simulink model "AFASClosedloopSim"  (R2023a)
settings: Solver=FixedStepAuto  StartTime=0.0  StopTime=600  FixedStep=1/240  RelTol=1e-5
PreLoadFcn:
  | [aircraft, state] = astDehavillandBeaver();
  | thrustX = getCoefficient(aircraft,"CX","Propeller",Component="Propeller");
InitFcn:
  | AFASClosedloopSimInitialization
model workspace (MATLAB code in the model file + MAT data in the model file):
  AirReferencedVelocity = 1
  AircraftPerformance : object (value not decoded)
  CurrentWaypoint = 1
  FCCLatDirMode = 1
  FCCVerticalMode = 1
  FlightPlan = 1
  LookaheadDis = 15
  NextWaypoint = 1
  NumofWaypoint = 1
  OwnshipAircraftID = 1
  PreWaypoint = 1
  PreviousWaypoint : Simulink.Parameter (value not decoded)
  TrajectoryChange = 1
  WaypointType = 1
  inputs0 : object (value not decoded)
  states : object (value not decoded)
  states0 : object (value not decoded)
  other statements: initialize6DOFSkyHogg;
values from neighbouring files (symbols this model uses):
  alt_ft = 1000    [AFASClosedloopSimInitialization.m]
  alt_hold_av = 1.5    [AFASClosedloopSimInitialization.m]
  alt_hold_hold = 0.1    [AFASClosedloopSimInitialization.m]
  alt_hold_vs = 0.58    [AFASClosedloopSimInitialization.m]
  alt_m = 304.8    [AFASClosedloopSimInitialization.m]
  AT_lead_T1 = 1    [AFASClosedloopSimInitialization.m]
  AT_lead_T2 = 1    [AFASClosedloopSimInitialization.m]
  AT_spd_hold_cmpst = 0.5    [AFASClosedloopSimInitialization.m]
  AT_spd_hold_ptch_tau_gain = 0.15    [AFASClosedloopSimInitialization.m]
  AT_spd_hold_rate_damping_gain = 10    [AFASClosedloopSimInitialization.m]
  AT_spd_hold_tas_lp_tau = 5.0    (= 5)    [AFASClosedloopSimInitialization.m]
  AT_spd_hold_tas_val_lp_tau = 0.5    [AFASClosedloopSimInitialization.m]
  AT_struct_den = 1    [AFASClosedloopSimInitialization.m]
  AT_struct_num = 1    [AFASClosedloopSimInitialization.m]
  AT_svo_composite = 1    [AFASClosedloopSimInitialization.m]
  av_hp_fltr_tau = 10    [AFASClosedloopSimInitialization.m]
  av_lp_fltr_tau = 0.5    [AFASClosedloopSimInitialization.m]
  cas_mps = 72.0222    [AFASClosedloopSimInitialization.m]
  Cl0 = 5.910000000000000e-04    (= 0.000591)    [AFASClosedloopSimInitialization.m]
  Cl_beta = -0.0618    [AFASClosedloopSimInitialization.m]
  Cl_da = -0.0992    [AFASClosedloopSimInitialization.m]
  Cl_da_alpha = -0.0827    [AFASClosedloopSimInitialization.m]
  Cl_dr = 0.0069    [AFASClosedloopSimInitialization.m]
  Cl_p = -0.5045    [AFASClosedloopSimInitialization.m]
  Cl_r = 0.1695    [AFASClosedloopSimInitialization.m]
  Cm0 = 0.0945    [AFASClosedloopSimInitialization.m]
  Cm_alpha = -0.6028    [AFASClosedloopSimInitialization.m]
  Cm_alpha2 = -2.1400    (= -2.14)    [AFASClosedloopSimInitialization.m]
  Cm_beta2 = 0.6921    [AFASClosedloopSimInitialization.m]
  Cm_de = -1.9210    (= -1.921)    [AFASClosedloopSimInitialization.m]
  Cm_df = 0.4072    [AFASClosedloopSimInitialization.m]
  Cm_q = -15.5600    (= -15.56)    [AFASClosedloopSimInitialization.m]
  Cm_r = -0.3118    [AFASClosedloopSimInitialization.m]
  Cn0 = -0.0031    [AFASClosedloopSimInitialization.m]
  Cn_beta = 0.0067    [AFASClosedloopSimInitialization.m]
  Cn_beta3 = 0.1373    [AFASClosedloopSimInitialization.m]
  Cn_da = -0.0039    [AFASClosedloopSimInitialization.m]
  Cn_dr = -0.0827    [AFASClosedloopSimInitialization.m]
  Cn_p = -0.1585    [AFASClosedloopSimInitialization.m]
  Cn_q = 0.1595    [AFASClosedloopSimInitialization.m]
  Cn_r = -0.1112    [AFASClosedloopSimInitialization.m]
  Cx0 = -0.0355    [AFASClosedloopSimInitialization.m]
  Cx_alpha = 0.0029    [AFASClosedloopSimInitialization.m]
  Cx_alpha2 = 5.4590    (= 5.459)    [AFASClosedloopSimInitialization.m]
  Cx_alpha3 = -5.1620    (= -5.162)    [AFASClosedloopSimInitialization.m]
  Cx_df = -0.0945    [AFASClosedloopSimInitialization.m]
  Cx_df_alpha = 1.1060    (= 1.106)    [AFASClosedloopSimInitialization.m]
  Cx_dr = 0.0341    [AFASClosedloopSimInitialization.m]
  Cx_q = -0.6748    [AFASClosedloopSimInitialization.m]
  Cy0 = -0.0022    [AFASClosedloopSimInitialization.m]
  Cy_beta = -0.7678    [AFASClosedloopSimInitialization.m]
  Cy_da = -0.0296    [AFASClosedloopSimInitialization.m]
  Cy_dr = 0.1158    [AFASClosedloopSimInitialization.m]
  Cy_dr_alpha = 0.5238    [AFASClosedloopSimInitialization.m]
  Cy_p = -0.1240    (= -0.124)    [AFASClosedloopSimInitialization.m]
  Cy_r = 0.3666    [AFASClosedloopSimInitialization.m]
  Cz0 = -0.0550    (= -0.055)    [AFASClosedloopSimInitialization.m]
  Cz_alpha = -5.5780    (= -5.578)    [AFASClosedloopSimInitialization.m]
  Cz_alpha3 = 3.4420    (= 3.442)    [AFASClosedloopSimInitialization.m]
  Cz_de = -0.3980    (= -0.398)    [AFASClosedloopSimInitialization.m]
  Cz_de_beta = -15.9300    (= -15.93)    [AFASClosedloopSimInitialization.m]
  Cz_df = -1.3770    (= -1.377)    [AFASClosedloopSimInitialization.m]
  Cz_df_alpha = -1.2610    (= -1.261)    [AFASClosedloopSimInitialization.m]
  Cz_q = -2.9880    (= -2.988)    [AFASClosedloopSimInitialization.m]
  hdg_select_hdg_rate_capt = 0.2    [AFASClosedloopSimInitialization.m]
  hdg_select_hdg_rate_damping = 1    [AFASClosedloopSimInitialization.m]
  hdg_select_hdg_rate_track = 0.05    [AFASClosedloopSimInitialization.m]
  lat_accel_aug_lp_tau = 10    [AFASClosedloopSimInitialization.m]
  ltrl_acc_gain = -0.04    [AFASClosedloopSimInitialization.m]
  ltrl_acc_lp_tau = 0.5    [AFASClosedloopSimInitialization.m]
  mach = 0.213    [AFASClosedloopSimInitialization.m]
  OwnshipAircraftConfig = 0    [AFASClosedloopSimInitialization.m]
  pitch_att_gain = 0.7    [AFASClosedloopSimInitialization.m]
  pitch_lead_T1 = 1    [AFASClosedloopSimInitialization.m]
  pitch_lead_T2 = 1    [AFASClosedloopSimInitialization.m]
  pitch_rate_gain = -1400    [AFASClosedloopSimInitialization.m]
  pitch_rate_gain_GAIN1 = -56    [AFASClosedloopSimInitialization.m]
  pitch_rate_gain_GAIN2 = -52.25    [AFASClosedloopSimInitialization.m]
  pitch_rate_gain_IAS1 = 100    [AFASClosedloopSimInitialization.m]
  pitch_rate_gain_IAS2 = 380    [AFASClosedloopSimInitialization.m]
  pitch_rate_gain_schd = [4.24        2.80        2.24        1.68        1.44        1.22        0.97        0.85        0.77        0.72        0.66    ] * 1000    [AFASClosedloopSimInitialization.m]
  pitch_rate_gain_spd = [85          100.0       120.00      140.00      160.00      180.00      200.00      220.00      240.00      260.00      275.00  ] * 0.5144444    [AFASClosedloopSimInitialization.m]
  pitch_schedule_type = 3    [AFASClosedloopSimInitialization.m]
  pitch_struct_den = 1    [AFASClosedloopSimInitialization.m]
  pitch_struct_num = 1    [AFASClosedloopSimInitialization.m]
  pitch_svo_composite = 1    [AFASClosedloopSimInitialization.m]
  pitch_svo_integral = 0.6    [AFASClosedloopSimInitialization.m]
  roll_att_gain = 0.45    [AFASClosedloopSimInitialization.m]
  roll_lead_T1 = 1    [AFASClosedloopSimInitialization.m]
  roll_lead_T2 = 1    [AFASClosedloopSimInitialization.m]
  roll_limit = 30*d2r    (= 0.5235987)    [AFASClosedloopSimInitialization.m]
  roll_rate_gain = 561.5    [AFASClosedloopSimInitialization.m]
  roll_rate_gain_GAIN1 = 57.25    [AFASClosedloopSimInitialization.m]
  roll_rate_gain_GAIN2 = 41.25    [AFASClosedloopSimInitialization.m]
  roll_rate_gain_IAS1 = 100    [AFASClosedloopSimInitialization.m]
  roll_rate_gain_IAS2 = 380    [AFASClosedloopSimInitialization.m]
  roll_rate_gain_schd = [1.30        0.86        0.71        0.63        0.57        0.50        0.46        0.46    ] * 1000    [AFASClosedloopSimInitialization.m]
  roll_rate_gain_spd = [85.00       100.00      120.00      140.00      160.00      200.00      220.00      275.00  ] * 0.5144444    [AFASClosedloopSimInitialization.m]
  roll_schedule_type = 3    [AFASClosedloopSimInitialization.m]
  roll_struct_den = 1    [AFASClosedloopSimInitialization.m]
  roll_struct_num = 1    [AFASClosedloopSimInitialization.m]
  roll_svo_composite = 0.00001    (= 1e-05)    [AFASClosedloopSimInitialization.m]
  roll_svo_integral = 0.6    [AFASClosedloopSimInitialization.m]
  tas_mps = 73.051    [AFASClosedloopSimInitialization.m]
  TGR = 0.25    [AFASClosedloopSimInitialization.m]
  wingrock_enable_alt = 20000    [AFASClosedloopSimInitialization.m]
  wingrock_enable_mach = 0.6    [AFASClosedloopSimInitialization.m]
  wingrock_lookup_data = [2 2  1 1]    [AFASClosedloopSimInitialization.m]
  wingrock_lookup_row = [0 2 5 10]*pi/180    [AFASClosedloopSimInitialization.m]
  wingrock_schedule_type = 3    [AFASClosedloopSimInitialization.m]
  yaw_rate_gain = 15521    [AFASClosedloopSimInitialization.m]
  yaw_rate_gain_GAIN1 = 37.8352    [AFASClosedloopSimInitialization.m]
  yaw_rate_gain_GAIN2 = 24.2654    [AFASClosedloopSimInitialization.m]
  yaw_rate_gain_IAS1 = 100    [AFASClosedloopSimInitialization.m]
  yaw_rate_gain_IAS2 = 340    [AFASClosedloopSimInitialization.m]
  yaw_rate_gain_piecewise_schd = [7.68	5.98		3.22	2.59		1.78 ... (first row only)    [AFASClosedloopSimInitialization.m]
  yaw_rate_gain_schd = [15521    11532   11532   10115   8951.7  7831.7  6829.2  5739.3  4506.7  3317.9  3391.5  2103.9  1404.5  994.3226]    [AFASClosedloopSimInitialization.m]
  yaw_rate_gain_spd = [90       97      106     111     118     127     136     149     165     187     192     228     264     295     ] * 0.5144444    [AFASClosedloopSimInitialization.m]
  yaw_rate_hp_tau = 1.8    [AFASClosedloopSimInitialization.m]
  yd_lead_T1 = yd_a * yd_lead_T2    [AFASClosedloopSimInitialization.m]
  ... (+7 more)
undefined symbols (not defined in the file or in its folder): aircraft, DiscIntNeverNeededParam, Earth, F, Light, MIL, sigbuilder_block, state, WGS84
libraries: aerolibasang x4, aerolibactuator x4, aerolibguid x2, simulink x2, dspnetwork x2, etargetslib x2, shared6dof x1, aerolibadyn x1, aerolibatmos2 x1, aerolibwind2 x1, aerolibtransform2 x1, sharedtransform x1
(part 3 of 4)

== system AFASClosedloopSim/FMGC (Flight Mgt and Guidance & Control)/AFCC: Albatross.ai Flight Control Computer/FCC: Outerloop & Innerloop Control Laws ==
  SpdTargetLimited : Inport
  AltTargetLimited : Inport  Port=2
  HDGTargetLimited : Inport  Port=3
  OwnshipStates : Inport  Port=4
  ALT Mode : Subsystem
  Autothrottle : Subsystem
  HDG Mode : Subsystem
  ATServoCmd : Outport
  PitchServoCmd : Outport  Port=2
  RollSevoCmd : Outport  Port=3
  YawServoCmd : Outport  Port=4
  wires:
  Autothrottle/1(ATServoCmd) -> ATServoCmd/1
  SpdTargetLimited/1 -> Autothrottle/1(SpeedTargetLimited)
  AltTargetLimited/1 -> ALT Mode/1(AltTargetLimited)
  OwnshipStates/1 -> HDG Mode/2(OwnshipStates), ALT Mode/2(OwnshipStates), Autothrottle/2(OwnshipStates)
  HDGTargetLimited/1 -> HDG Mode/1(HDGTargetLimited)
  ALT Mode/1(motorPosCmd_rad) -> PitchServoCmd/1
  HDG Mode/1(ailMotorPosCmd_rad) -> RollSevoCmd/1
  HDG Mode/2(rudMotorPosCmd_rad) -> YawServoCmd/1

== system AFASClosedloopSim/FMGC (Flight Mgt and Guidance & Control)/AFMS: Albatross Flight Management System/WGS84_Location ==
  lon : Inport
  lat : Inport  Port=2
  alt : Inport  Port=3
  C Caller : CCaller  FunctionName=latToMeters  PortSpecificationStruct="%)30     .    6 4   8    (     @         %    \"     ,    !     0         %  0 \"0    $    _    07)G3F%M90  4&]R=$YA;64 4V-O<&4     26YD97@     5'EP90      4VEZ90      27-';&]B86P   X    P    !@    @    $          4    (     0    ,    !         !   P!O=70 #@   #     &    \"     0         !0    @    !     P    $         $  # &]U=  .    .     8    (    !          %    \"     $    &     0         0    !@   $]U='!U=   #@   #@    &    \"     8         !0    @    !     0    $         \"0    @               X    X    !@    @    $          4    (     0    8    !         !     &    9&]U8FQE   .    ,     8    (    !          %    \"     $    !     0         0  $ ,0    X    P    !@    @    ) @        4    (     0    $    !          (  0      #@   #     &    \"     0         !0    @    !    !     $         $  $ &QA=#$.    ,     8    (    !          %    \"     $    $     0         0  0 ;&%T,0X    X    !@    @    $          4    (     0    4    !         !     %    26YP=70    .    .     8    (    !@         %    \"     $    !     0         )    \"               #@   #@    &    \"     0         !0    @    !    !@    $         $     8   !D;W5B;&4   X    P    !@    @    $          4    (     0    $    !         !   0 Q    #@   #     &    \"     D\"        !0    @    !     0    $          @ !       .    ,     8    (    !          %    \"     $    $     0         0  0 ;&%T,@X    P    !@    @    $          4    (     0    0    !         !  ! !L870R#@   #@    &    \"     0         !0    @    !    !0    $         $     4   !);G!U=     X    X    !@    @    &          4    (     0    $    !          D    (            \\#\\.    .     8    (    !          %    \"     $    &     0         0    !@   &1O=6)L90  #@   #     &    \"     0         !0    @    !     0    $         $  ! #$    .    ,     8    (    \"0(        %    \"     $    !     0         \"  $"
  C Caller1 : CCaller  FunctionName=lonToMeters  PortSpecificationStruct="%)30     .    ^ 8   8    (     @         %    \"     0    !     0         %  0 \"0    $    _    07)G3F%M90  4&]R=$YA;64 4V-O<&4     26YD97@     5'EP90      4VEZ90      27-';&]B86P   X    P    !@    @    $          4    (     0    ,    !         !   P!O=70 #@   #     &    \"     0         !0    @    !     P    $         $  # &]U=  .    .     8    (    !          %    \"     $    &     0         0   ...(+2020 chars)"
  lat1 : Constant  Value=39.13730579607521
  lon1 : Constant  Value=117.33825437858884
  x : Outport
  y : Outport  Port=2
  z : Outport  Port=3
  wires:
  lon1/1 -> C Caller1/2
  lon/1 -> C Caller1/1
  alt/1 -> z/1
  lat1/1 -> C Caller/2, C Caller1/3
  lat/1 -> C Caller/1
  C Caller/1 -> y/1
  C Caller1/1 -> x/1

== system AFASClosedloopSim/6 DoF Airframe Model/Aerodynamic Model/Actuator Increments/Aileron ==
  alpha : Inport  Unit=rad
  Actuators : Inport  Port=2  Unit=rad
  Gain1 : Gain  Gain=0  SaturateOnIntegerOverflow=on  OutDataTypeStr=Inherit: Same as input  ParamDataTypeStr=Inherit: Same as input
  Gain2 : Gain  Gain=Cy_da  SaturateOnIntegerOverflow=on  OutDataTypeStr=Inherit: Same as input  ParamDataTypeStr=Inherit: Same as input
  Gain3 : Gain  Gain=0  SaturateOnIntegerOverflow=on  OutDataTypeStr=Inherit: Same as input  ParamDataTypeStr=Inherit: Same as input
  Gain4 : Gain  Gain=Cn_da  SaturateOnIntegerOverflow=on  OutDataTypeStr=Inherit: Same as input  ParamDataTypeStr=Inherit: Same as input
  Gain5 : Gain  Gain=0  SaturateOnIntegerOverflow=on  OutDataTypeStr=Inherit: Same as input  ParamDataTypeStr=Inherit: Same as input
  Gain6 : Gain  Gain=Cl_da  SaturateOnIntegerOverflow=on  OutDataTypeStr=Inherit: Same as input  ParamDataTypeStr=Inherit: Same as input
  Gain7 : Gain  Gain=Cl_da_alpha  SaturateOnIntegerOverflow=on  OutDataTypeStr=Inherit: Same as input  ParamDataTypeStr=Inherit: Same as input
  Mux1 : Mux  Inputs=6
  Product4 : Product  InputSameDT=on  SaturateOnIntegerOverflow=on  OutDataTypeStr=Inherit: Same as first input
  Selector1 : Selector  IndexMode=Zero-based  InputPortWidth=4  IndexOptions=Index vector (dialog)  Indices=1  OutputSizes=1
  Sum1 : Sum  Inputs=++|  SaturateOnIntegerOverflow=on
  delCoeff : Outport  VectorParamsAs1DForOutWhenUnconnected=off
  wires:
  Gain6/1 -> Sum1/1
  Sum1/1 -> Mux1/4
  Gain7/1 -> Sum1/2
  Product4/1 -> Gain7/1
  Gain1/1 -> Mux1/1  "Cx"
  alpha/1 -> Product4/2
  Actuators/1 -> Selector1/1
  Mux1/1 -> delCoeff/1
  Gain2/1 -> Mux1/2  "Cy"
  Gain3/1 -> Mux1/3  "Cz"
  Gain5/1 -> Mux1/5  "Cm"
  Gain4/1 -> Mux1/6
  Selector1/1 -> Gain1/1, Gain2/1, Gain3/1, Gain6/1, Product4/1, Gain5/1, Gain4/1

== system AFASClosedloopSim/6 DoF Airframe Model/Aerodynamic Model/Actuator Increments/Elevator ==
  Actuators : Inport
  Beta : Inport  Port=2  Unit=rad
  Constant1 : Constant  Value=0
  Gain1 : Gain  Gain=Cz_de  SaturateOnIntegerOverflow=on  OutDataTypeStr=Inherit: Same as input  ParamDataTypeStr=Inherit: Same as input
  Gain2 : Gain  Gain=Cz_de_beta  SaturateOnIntegerOverflow=on  OutDataTypeStr=Inherit: Same as input  ParamDataTypeStr=Inherit: Same as input
  Gain3 : Gain  Gain=Cm_de  SaturateOnIntegerOverflow=on  OutDataTypeStr=Inherit: Same as input  ParamDataTypeStr=Inherit: Same as input
  Mux1 : Mux  Inputs=6
  Product4 : Product  Inputs=3  InputSameDT=on  SaturateOnIntegerOverflow=on  OutDataTypeStr=Inherit: Same as first input
  Selector1 : Selector  IndexMode=Zero-based  InputPortWidth=4  IndexOptions=Index vector (dialog)  Indices=0  OutputSizes=1
  Sum1 : Sum  SaturateOnIntegerOverflow=on
  delCoeff : Outport  VectorParamsAs1DForOutWhenUnconnected=off
  wires:
  Gain3/1 -> Mux1/5
  Gain1/1 -> Sum1/2
  Gain2/1 -> Sum1/1
  Sum1/1 -> Mux1/3
  Product4/1 -> Gain2/1
  Beta/1 -> Product4/2, Product4/1
  Mux1/1 -> delCoeff/1
  Selector1/1 -> Gain3/1, Gain1/1, Product4/3
  Constant1/1 -> Mux1/1, Mux1/2, Mux1/4, Mux1/6
  Actuators/1 -> Selector1/1

== system AFASClosedloopSim/6 DoF Airframe Model/Aerodynamic Model/Actuator Increments/Flap ==
  Alpha : Inport  Unit=rad
  Actuators : Inport  Port=2  Unit=rad
  Constant1 : Constant  Value=0
  Constant2 : Constant  Value=0
  Constant3 : Constant  Value=0
  Gain1 : Gain  Gain=Cx_df  SaturateOnIntegerOverflow=on  OutDataTypeStr=Inherit: Same as input  ParamDataTypeStr=Inherit: Same as input
  Gain2 : Gain  Gain=Cx_df_alpha  SaturateOnIntegerOverflow=on  OutDataTypeStr=Inherit: Same as input  ParamDataTypeStr=Inherit: Same as input
  Gain3 : Gain  Gain=Cz_df  SaturateOnIntegerOverflow=on  OutDataTypeStr=Inherit: Same as input  ParamDataTypeStr=Inherit: Same as input
  Gain4 : Gain  Gain=Cz_df_alpha  SaturateOnIntegerOverflow=on  OutDataTypeStr=Inherit: Same as input  ParamDataTypeStr=Inherit: Same as input
  Gain5 : Gain  Gain=Cm_df  SaturateOnIntegerOverflow=on  OutDataTypeStr=Inherit: Same as input  ParamDataTypeStr=Inherit: Same as input
  Mux1 : Mux  Inputs=6
  Product1 : Product  InputSameDT=on  SaturateOnIntegerOverflow=on  OutDataTypeStr=Inherit: Same as first input
  Product4 : Product  InputSameDT=on  SaturateOnIntegerOverflow=on  OutDataTypeStr=Inherit: Same as first input
  Selector1 : Selector  IndexMode=Zero-based  InputPortWidth=4  IndexOptions=Index vector (dialog)  Indices=3  OutputSizes=1
  Sum1 : Sum  SaturateOnIntegerOverflow=on
  Sum2 : Sum  SaturateOnIntegerOverflow=on
  delCoeff : Outport  VectorParamsAs1DForOutWhenUnconnected=off
  wires:
  Selector1/1 -> Gain1/1, Product4/1, Product1/1, Gain3/1, Gain5/1
  Actuators/1 -> Selector1/1
  Gain5/1 -> Mux1/5
  Gain3/1 -> Sum2/1
  Gain4/1 -> Sum2/2
  Product1/1 -> Gain4/1
  Gain1/1 -> Sum1/1
  Gain2/1 -> Sum1/2
  Product4/1 -> Gain2/1
  Alpha/1 -> Product1/2, Product4/2
  Mux1/1 -> delCoeff/1
  Sum1/1 -> Mux1/1
  Sum2/1 -> Mux1/3
  Constant1/1 -> Mux1/2
  Constant2/1 -> Mux1/4
  Constant3/1 -> Mux1/6

== system AFASClosedloopSim/6 DoF Airframe Model/Aerodynamic Model/Actuator Increments/Rudder ==
  Alpha : Inport  Unit=rad
  Actuators : Inport  Port=2  Unit=rad
  Constant1 : Constant  Value=0
  Constant2 : Constant  Value=0
  Gain1 : Gain  Gain=Cl_dr  SaturateOnIntegerOverflow=on  OutDataTypeStr=Inherit: Same as input  ParamDataTypeStr=Inherit: Same as input
  Gain2 : Gain  Gain=Cn_dr  SaturateOnIntegerOverflow=on  OutDataTypeStr=Inherit: Same as input  ParamDataTypeStr=Inherit: Same as input
  Gain3 : Gain  Gain=Cy_dr_alpha  SaturateOnIntegerOverflow=on  OutDataTypeStr=Inherit: Same as input  ParamDataTypeStr=Inherit: Same as input
  Gain4 : Gain  Gain=Cy_dr  SaturateOnIntegerOverflow=on  OutDataTypeStr=Inherit: Same as input  ParamDataTypeStr=Inherit: Same as input
  Gain5 : Gain  Gain=Cx_dr  SaturateOnIntegerOverflow=on  OutDataTypeStr=Inherit: Same as input  ParamDataTypeStr=Inherit: Same as input
  Mux1 : Mux  Inputs=6
  Product1 : Product  InputSameDT=on  SaturateOnIntegerOverflow=on  OutDataTypeStr=Inherit: Same as first input
  Selector1 : Selector  IndexMode=Zero-based  InputPortWidth=4  IndexOptions=Index vector (dialog)  Indices=2  OutputSizes=1
  Sum1 : Sum  SaturateOnIntegerOverflow=on
  delCoeff : Outport  VectorParamsAs1DForOutWhenUnconnected=off
  wires:
  Gain5/1 -> Mux1/1
  Gain4/1 -> Sum1/1
  Gain3/1 -> Sum1/2
  Gain1/1 -> Mux1/4
  Gain2/1 -> Mux1/6
  Product1/1 -> Gain3/1
  Alpha/1 -> Product1/2
  Mux1/1 -> delCoeff/1
  Actuators/1 -> Selector1/1
  Sum1/1 -> Mux1/2
  Constant1/1 -> Mux1/3
  Constant2/1 -> Mux1/5
  Selector1/1 -> Gain5/1, Gain4/1, Product1/1, Gain1/1, Gain2/1

== system AFASClosedloopSim/6 DoF Airframe Model/Aerodynamic Model/Body Rate Damping/p ==
  Constant1 : Constant  Value=0
  Constant2 : Constant  Value=Cy_p
  Constant3 : Constant  Value=Cl_p
  Constant4 : Constant  Value=Cn_p
  Mux1 : Mux  Inputs=6
  delCoeff : Outport  VectorParamsAs1DForOutWhenUnconnected=off
  wires:
  Constant2/1 -> Mux1/2
  Mux1/1 -> delCoeff/1
  Constant1/1 -> Mux1/5, Mux1/3, Mux1/1
  Constant4/1 -> Mux1/6
  Constant3/1 -> Mux1/4

== system AFASClosedloopSim/6 DoF Airframe Model/Aerodynamic Model/Body Rate Damping/q ==
  Constant1 : Constant  Value=0
  Constant2 : Constant  Value=Cz_q
  Constant3 : Constant  Value=Cx_q
  Constant4 : Constant  Value=Cm_q
  Constant5 : Constant  Value=Cn_q
  Mux1 : Mux  Inputs=6
  delCoeff : Outport  VectorParamsAs1DForOutWhenUnconnected=off
  wires:
  Constant2/1 -> Mux1/3
  Constant5/1 -> Mux1/6
  Constant1/1 -> Mux1/4, Mux1/2
  Constant4/1 -> Mux1/5
  Constant3/1 -> Mux1/1
  Mux1/1 -> delCoeff/1

== system AFASClosedloopSim/6 DoF Airframe Model/Aerodynamic Model/Body Rate Damping/r ==
  Constant : Constant  Value=0
  Constant1 : Constant  Value=Cy_r
  Constant2 : Constant  Value=Cl_r
  Constant3 : Constant  Value=Cm_r
  Constant4 : Constant  Value=Cn_r
  Mux1 : Mux  Inputs=6
  delCoeff : Outport  VectorParamsAs1DForOutWhenUnconnected=off
  wires:
  Constant3/1 -> Mux1/5
  Constant1/1 -> Mux1/2
  Constant4/1 -> Mux1/6
  Constant2/1 -> Mux1/4
  Constant/1 -> Mux1/3, Mux1/1
  Mux1/1 -> delCoeff/1

== system AFASClosedloopSim/FMGC (Flight Mgt and Guidance & Control)/AFCC: Albatross.ai Flight Control Computer/FCC: Outerloop & Innerloop Control Laws/ALT Mode ==
  AltTargetLimited : Inport
  OwnshipStates : Inport  Port=2
  ADC Filters & Delays : Subsystem
  AHRS Filters & Delays : Subsystem
  Bus Selector : BusSelector  OutputSignals=Ze,q
  Derivative : Derivative
  Derivative1 : Derivative
  Innerloop Control Law : Subsystem
  Outerloop Control Law : Subsystem
  motorPosCmd_rad : Outport
  wires:
  Outerloop Control Law/1(thetaCmd_rad) -> Innerloop Control Law/1("thetaCmd_rad ")
  Outerloop Control Law/2(" qC_rps ") -> Innerloop Control Law/2(qC_rps)
  ADC Filters & Delays/1(hF_m) -> Outerloop Control Law/2(hF_m)
  AltTargetLimited/1 -> Outerloop Control Law/1(hCmd_m)
  Innerloop Control Law/1(motorPosCmd_rad) -> motorPosCmd_rad/1
  AHRS Filters & Delays/2(qF_rps) -> Outerloop Control Law/5(qF_rps)
  ADC Filters & Delays/2(hdF_mps) -> Outerloop Control Law/3(hdF_mps)
  Derivative/1 -> Derivative1/1, ADC Filters & Delays/2(hd_mps)
  Bus Selector/1 -> ADC Filters & Delays/1(h_m), Derivative/1  "<Ze>"
  AHRS Filters & Delays/1(hddF_mpss) -> Outerloop Control Law/4(hddF_mpss)
  OwnshipStates/1 -> Bus Selector/1
  Derivative1/1 -> AHRS Filters & Delays/1(hdd_mpss)
  Bus Selector/2 -> AHRS Filters & Delays/2(qb_rps)  "<q>"

== system AFASClosedloopSim/FMGC (Flight Mgt and Guidance & Control)/AFCC: Albatross.ai Flight Control Computer/FCC: Outerloop & Innerloop Control Laws/Autothrottle ==
  SpeedTargetLimited : Inport
  OwnshipStates : Inport  Port=2
  ADC Filters & Delays : Subsystem
  AT Innerloop : Subsystem
  AT SPD Hold/Select : Subsystem
  Add : Sum  Inputs=+-
  Bus Selector : BusSelector  OutputSignals=u
  Constant : Constant
  Constant1 : Constant
  Manual Switch1 : ManualSwitch
  Manual Switch2 : ManualSwitch
  g2mpss2 : Gain  Gain=AT_svo_composite  SaturateOnIntegerOverflow=on  OutDataTypeStr=Inherit: Same as input  ParamDataTypeStr=Inherit: Same as input
  ATServoCmd : Outport
  wires:
  OwnshipStates/1 -> Bus Selector/1
  AT SPD Hold/Select/1(ATCmd_rad) -> AT Innerloop/1("ATCmd_rad ")
  ADC Filters & Delays/1(vtasF_mps) -> AT SPD Hold/Select/2(vtasF_mps)
  Bus Selector/1 -> Add/2  "<u>"
  Add/1 -> g2mpss2/1
  g2mpss2/1 -> Manual Switch1/1
  AT Innerloop/1(motorPosCmd_rad) -> Manual Switch1/2
  Manual Switch1/1 -> ATServoCmd/1
  SpeedTargetLimited/1 -> Manual Switch2/1
  Manual Switch2/1 -> Add/1
  Constant/1 -> AT SPD Hold/Select/1(vtasCmd_mps)
  Constant1/1 -> ADC Filters & Delays/1(vtas_mps)

== system AFASClosedloopSim/FMGC (Flight Mgt and Guidance & Control)/AFCC: Albatross.ai Flight Control Computer/FCC: Outerloop & Innerloop Control Laws/HDG Mode ==
  HDGTargetLimited : Inport
  OwnshipStates : Inport  Port=2
  Bus Selector : BusSelector  OutputSignals=psi,phi,r,Ayb
  Derivative : Derivative
  Derivative1 : Derivative
  Filters & Delays : Subsystem
  Innerloop Control Law : Subsystem
  Outerloop Control Law : Subsystem
  ailMotorPosCmd_rad : Outport
  rudMotorPosCmd_rad : Outport  Port=2
  wires:
  Outerloop Control Law/2(phiC_rad) -> Innerloop Control Law/2(phiC_rad)
  Filters & Delays/4(phiDotF_rps) -> Outerloop Control Law/5("phiDotF_rps ")
  Outerloop Control Law/3(rC_rps) -> Innerloop Control Law/3(rC_rps)
  Bus Selector/2 -> Derivative1/1, Filters & Delays/3(phi_rad)  "<phi>"
  Outerloop Control Law/4(AyC_mpss) -> Innerloop Control Law/4(AyC_mpss)
  Innerloop Control Law/2(rudMotorPosCmd_rad) -> rudMotorPosCmd_rad/1
  Outerloop Control Law/5(phiDotC_rps) -> Innerloop Control Law/5(phidotC_rps)
  Innerloop Control Law/1(ailMotorPosCmd_rad) -> ailMotorPosCmd_rad/1
  Filters & Delays/3(phiF_rad) -> Outerloop Control Law/4("phiF_rad ")
  HDGTargetLimited/1 -> Outerloop Control Law/1(psiCmd_rad)
  Filters & Delays/2(psiDotF_rps) -> Outerloop Control Law/3(psiDotF_rps)
  Filters & Delays/6(AyF_mpss) -> Outerloop Control Law/7("AyF_mpss ")
  Filters & Delays/1(psiF_rad) -> Outerloop Control Law/2(psiF_rad)
  Filters & Delays/5(rF_rps) -> Outerloop Control Law/6(rF_rps)
  Outerloop Control Law/1(phiCmd_rad) -> Innerloop Control Law/1(phiCmd_rad)
  OwnshipStates/1 -> Bus Selector/1
  Bus Selector/1 -> Derivative/1, Filters & Delays/1(psi_rad)  "<psi>"
  Derivative/1 -> Filters & Delays/2(psiDot_rps)
  Derivative1/1 -> Filters & Delays/4(phiDot_rps)
  Bus Selector/3 -> Filters & Delays/5(rb_rps)  "<r>"
  Bus Selector/4 -> Filters & Delays/6(AyAH_mpss)  "<Ayb>"

== system AFASClosedloopSim/FMGC (Flight Mgt and Guidance & Control)/AFCC: Albatross.ai Flight Control Computer/FCC: Outerloop & Innerloop Control Laws/ALT Mode/ADC Filters & Delays ==
  h_m : Inport
  hd_mps : Inport  Port=2
  ADC S/W and H/W Analog Filter Delay : TransportDelay  DelayTime=0.016
  ADC S/W and H/W Analog Filter Delay1 : TransportDelay  DelayTime=0.016
  AHRS ARINC429 Delay : TransportDelay  DelayTime=0.025082
  ARINC429 Delay : TransportDelay  DelayTime=0.022539
  H Anti-aliasing Filter : TransferFcn  Numerator=[0.005408 0.3963 5.095]  Denominator=[1 3.188 5.095]
  Hd Anti-aliasing Filter : TransferFcn  Numerator=[0.8436]  Denominator=[1 1.6533 0.8436]
  hF_m : Outport
  hdF_mps : Outport  Port=2
  wires:
  h_m/1 -> H Anti-aliasing Filter/1
  hd_mps/1 -> Hd Anti-aliasing Filter/1
  ADC S/W and H/W Analog Filter Delay1/1 -> AHRS ARINC429 Delay/1
  AHRS ARINC429 Delay/1 -> hdF_mps/1
  H Anti-aliasing Filter/1 -> ADC S/W and H/W Analog Filter Delay/1
  ADC S/W and H/W Analog Filter Delay/1 -> ARINC429 Delay/1
  ARINC429 Delay/1 -> hF_m/1
  Hd Anti-aliasing Filter/1 -> ADC S/W and H/W Analog Filter Delay1/1

== system AFASClosedloopSim/FMGC (Flight Mgt and Guidance & Control)/AFCC: Albatross.ai Flight Control Computer/FCC: Outerloop & Innerloop Control Laws/ALT Mode/AHRS Filters & Delays ==
  hdd_mpss : Inport
  qb_rps : Inport  Port=2
  AHRS Delay : TransportDelay  DelayTime=0.014
  AHRS Delay1 : TransportDelay  DelayTime=0.014
  ARINC Delay : TransportDelay  DelayTime=0.00945
  ARINC Delay1 : TransportDelay  DelayTime=0.00745
  Hdd Anti-aliasing Filter : TransferFcn  Numerator=[2020.20]  Denominator=[1 75.76 2020.20]
  Internal Filter1 : TransferFcn  Numerator=[35600]  Denominator=[1 377.36 35600]
      settings: AttributesFormatString=Internal Filter
  Q Anti-aliasing Filter : TransferFcn  Numerator=[10000]  Denominator=[1 200 10000]
  hddF_mpss : Outport
  qF_rps : Outport  Port=2
  wires:
  ARINC Delay1/1 -> qF_rps/1
  Internal Filter1/1 -> Q Anti-aliasing Filter/1
  Q Anti-aliasing Filter/1 -> AHRS Delay1/1
  hdd_mpss/1 -> Hdd Anti-aliasing Filter/1
  Hdd Anti-aliasing Filter/1 -> AHRS Delay/1
  qb_rps/1 -> Internal Filter1/1
  AHRS Delay/1 -> ARINC Delay/1
  ARINC Delay/1 -> hddF_mpss/1
  AHRS Delay1/1 -> ARINC Delay1/1

== system AFASClosedloopSim/FMGC (Flight Mgt and Guidance & Control)/AFCC: Albatross.ai Flight Control Computer/FCC: Outerloop & Innerloop Control Laws/ALT Mode/Innerloop Control Law ==
  "thetaCmd_rad " : Inport
  qC_rps : Inport  Port=2
  Attitude Gain : Gain  Gain=pitch_att_gain  SaturateOnIntegerOverflow=on  OutDataTypeStr=Inherit: Same as input  ParamDataTypeStr=Inherit: Same as input
      settings: AttributesFormatString=%<Gain>
  Autopilot IAS-scheduled Gain : Subsystem  mask(Autopilot IAS-scheduled Gain){IAS1=pitch_rate_gain_IAS1, IAS2=pitch_rate_gain_IAS2, GAIN1=pitch_rate_gain_GAIN1, GAIN2=pitch_rate_gain_GAIN2}
      mask prompts: IAS1 "IAS1 (lower IAS limit, knots)"; IAS2 "IAS2 (upper IAS limit, knots)"; GAIN1 "GAIN1 (the gain for IAS1, dB)"; GAIN2 "GAIN2 (the gain for IAS2, dB)"
      mask help:
      | Autopilot gain scheduling based on the indicated airspeed.
      |
      | Parameters:
      | IAS1 (lower IAS limit, knots)  -- lower IAS limit (unit: knot)
      | IAS2 (upper IAS limit, knots) -- upper IAS limit (unit: knot)
      | GAIN1 (the gain for IAS1, dB) -- the gain for the lower IAS limit (unit: dB)
      | GAIN2 (the gain for IAS2, dB) -- the gain for the upper IAS limit (unit: dB)
      |
      | Inputs:
      | ias -- indicated airspeed (unit: meter/second)
      |
      | Outputs:
      | scheduled_gain -- indicated airspeed scheduled gain
      mask init:
      | ias_1 = IAS1 * 0.5144444;
      | ias_2 = IAS2 * 0.5144444;
      | abs_gain_1 = abs( GAIN1 ) * 8 / 6;
      | abs_gain_2 = abs( GAIN2 ) * 8 / 6;
      | gain_sign = sign( GAIN1 );
      mask Help:
      | Autopilot gain scheduling based on the indicated airspeed.
      | 
      | Parameters:
      | IAS1 (lower IAS limit, knots)  -- lower IAS limit (unit: knot)
      | IAS2 (upper IAS limit, knots) -- upper IAS limit (unit: knot)
      | GAIN1 (the gain for IAS1, dB) -- the gain for the lower IAS limit (unit: dB)
      | GAIN2 (the gain for IAS2, dB) -- the gain for the upper IAS limit (unit: dB)
      | 
      | Inputs:
      | ias -- indicated airspeed (unit: meter/second)
      | 
      | Outputs:
      | scheduled_gain -- indicated airspeed scheduled gain
  Constant1 : Constant  Value=cas_mps
      settings: AttributesFormatString=CAS_mps
  Display : Display
  Innerloop AP Delay : TransportDelay  DelayTime=0.003
  Integrator1 : Integrator
  Lead-Lag : TransferFcn  Numerator=[pitch_lead_T1 1]  Denominator=[pitch_lead_T2 1]
  Look-Up Table : Lookup  InputValues=pitch_rate_gain_spd  Table=pitch_rate_gain_schd  LookUpMeth=Interpolation-Use End Values
  Multiport Switch : MultiPortSwitch  InputSameDT=off
  Product1 : Product  Inputs=**  InputSameDT=on  SaturateOnIntegerOverflow=on  OutDataTypeStr=Inherit: Same as first input
  Structural Mode Filter3 : TransferFcn  Numerator=pitch_struct_num  Denominator=pitch_struct_den
  Sum1 : Sum  Inputs=-+|  SaturateOnIntegerOverflow=on
  Sum3 : Sum  Inputs=|++  SaturateOnIntegerOverflow=on
  g2mpss1 : Gain  Gain=pitch_svo_integral  SaturateOnIntegerOverflow=on  OutDataTypeStr=Inherit: Same as input  ParamDataTypeStr=Inherit: Same as input
  g2mpss2 : Gain  Gain=pitch_svo_composite  SaturateOnIntegerOverflow=on  OutDataTypeStr=Inherit: Same as input  ParamDataTypeStr=Inherit: Same as input
  schedule1 : Constant  Value=pitch_rate_gain
      settings: AttributesFormatString=pitch_rate_gain
  schedule_type : Constant  Value=pitch_schedule_type
  motorPosCmd_rad : Outport  InitialOutput=0
  wires:
  Sum1/1 -> Product1/1
  Constant1/1 -> Autopilot IAS-scheduled Gain/1(ias), Look-Up Table/1
  schedule1/1 -> Multiport Switch/2
  Look-Up Table/1 -> Multiport Switch/3
  Autopilot IAS-scheduled Gain/1(scheduled_gain) -> Multiport Switch/4
  schedule_type/1 -> Multiport Switch/1
  Multiport Switch/1 -> Product1/2, Display/1
  Attitude Gain/1 -> Sum1/2
  Integrator1/1 -> Sum3/2
  g2mpss1/1 -> Integrator1/1
  Sum3/1 -> g2mpss2/1
  Product1/1 -> Sum3/1, g2mpss1/1  "motorCmd_rps"
  "thetaCmd_rad "/1 -> Attitude Gain/1
  Structural Mode Filter3/1 -> Innerloop AP Delay/1
  Lead-Lag/1 -> Structural Mode Filter3/1
  g2mpss2/1 -> Lead-Lag/1
  qC_rps/1 -> Sum1/1
  Innerloop AP Delay/1 -> motorPosCmd_rad/1

== system AFASClosedloopSim/FMGC (Flight Mgt and Guidance & Control)/AFCC: Albatross.ai Flight Control Computer/FCC: Outerloop & Innerloop Control Laws/ALT Mode/Outerloop Control Law ==
  note: FPM to mps
  hCmd_m : Inport
  hF_m : Inport  Port=2
  hdF_mps : Inport  Port=3
  hddF_mpss : Inport  Port=4
  qF_rps : Inport  Port=5
  Alt Upset_m : Subsystem  Tag=STV Subsys  LoadFcn=sigbuilder_block('load');  StartFcn=sigbuilder_block('start');  StopFcn=sigbuilder_block('stop');  ClipboardFcn=sigbuilder_block('clipboard');  mask(Sigbuilder block){tuvar=[0:10]}
      mask help: Sigbuilder GUI
      mask init:
      | if ~strcmp(get_param(bdroot(gcbh),'SimulationStatus'),'stopped') tuvar = sigbuilder_block('maskInit'); end
      settings: CopyFcn=sigbuilder_block('copy');  DeleteFcn=sigbuilder_block('delete');  ModelCloseFcn=sigbuilder_block('modelClose');  PreSaveFcn=sigbuilder_block('preSave');  PauseFcn=sigbuilder_block('pause')  ContinueFcn=sigbuilder_block('continue')  NameChangeFcn=sigbuilder_block('namechange');  OpenFcn=sigbuilder_block('open',[154.5 129 653.25 399 ]);  CloseFcn=sigbuilder_block('close');
      mask Display: plot(0, 0, 100, 100,[2, 2, 32, 32, 2], [68, 8, 8, 68, 68],[32, 2], [38, 38], [32, 19, 2],[53, 60, 44], [32, 17, 17, 2],[16, 16, 31, 31]);txt = getActiveGroup(gcbh);text(2, 100, txt,'verticalAlignment', 'top');
  Attitude Gain1 : Gain  Gain=1/tas_mps  SaturateOnIntegerOverflow=on  OutDataTypeStr=Inherit: Same as input  ParamDataTypeStr=Inherit: Same as input
      settings: AttributesFormatString=%<Gain>
  Av_LP : TransferFcn  Denominator=[av_lp_fltr_tau 1]
  Complementary Filter : Subsystem
  Gain2 : Gain  Gain=0.00508
  Ground1 : Ground
  Ground2 : Ground
  Hold Gain : Gain  Gain=alt_hold_hold  SaturateOnIntegerOverflow=on  OutDataTypeStr=Inherit: Same as input  ParamDataTypeStr=Inherit: Same as input
      settings: AttributesFormatString=%<Gain>
  Manual Switch1 : ManualSwitch
  Manual Switch3 : ManualSwitch
  Outerloop AP Delay : TransportDelay  DelayTime=0.004
  Outerloop FD Delay : TransportDelay  DelayTime=0.0905
  PFD/MFD Delay : TransportDelay  DelayTime=0.030
  PFD/MFD Delay1 : TransportDelay  DelayTime=0.030
  PFD/MFD Delay2 : TransportDelay  DelayTime=0.0175
  Subsystem : Subsystem  mask(Zero-Order Hold){Tau=0.100}
      mask prompts: Tau "Tau (s)"
      mask help: Zero-Order Hold
      settings: AttributesFormatString=ZOH\n
      mask Display: disp([num2str(1/Tau),'Hz'])
  Subsystem1 : Subsystem  mask(Zero-Order Hold){Tau=0.025}
      mask prompts: Tau "Tau (s)"
      mask help: Zero-Order Hold
      settings: AttributesFormatString=ZOH\n
      mask Display: disp([num2str(1/Tau),'Hz'])
  Sum1 : Sum  Inputs=|+-  InputSameDT=on  SaturateOnIntegerOverflow=on  OutDataTypeStr=Inherit: Same as first input
  Sum2 : Sum  Inputs=++|  SaturateOnIntegerOverflow=on
  Sum3 : Sum  Inputs=|+-  SaturateOnIntegerOverflow=on
  Sum4 : Sum  Inputs=++|  SaturateOnIntegerOverflow=on
  Sum5 : Sum  Inputs=|+-  SaturateOnIntegerOverflow=on
  VS Gain : Gain  Gain=alt_hold_vs  SaturateOnIntegerOverflow=on  OutDataTypeStr=Inherit: Same as input  ParamDataTypeStr=Inherit: Same as input
      settings: AttributesFormatString=%<Gain>
  VS Upset_fpm : Subsystem  Tag=STV Subsys  LoadFcn=sigbuilder_block('load');  StartFcn=sigbuilder_block('start');  StopFcn=sigbuilder_block('stop');  ClipboardFcn=sigbuilder_block('clipboard');  mask(Sigbuilder block){tuvar=[0:10]}
      mask help: Sigbuilder GUI
      mask init:
      | if ~strcmp(get_param(bdroot(gcbh),'SimulationStatus'),'stopped') tuvar = sigbuilder_block('maskInit'); end
      settings: CopyFcn=sigbuilder_block('copy');  DeleteFcn=sigbuilder_block('delete');  ModelCloseFcn=sigbuilder_block('modelClose');  PreSaveFcn=sigbuilder_block('preSave');  PauseFcn=sigbuilder_block('pause')  ContinueFcn=sigbuilder_block('continue')  NameChangeFcn=sigbuilder_block('namechange');  OpenFcn=sigbuilder_block('open',[154.5 129 653.25 399 ]);  CloseFcn=sigbuilder_block('close');
      mask Display: plot(0, 0, 100, 100,[2, 2, 32, 32, 2], [68, 8, 8, 68, 68],[32, 2], [38, 38], [32, 19, 2],[53, 60, 44], [32, 17, 17, 2],[16, 16, 31, 31]);txt = getActiveGroup(gcbh);text(2, 100, txt,'verticalAlignment', 'top');
  Vertical Accel Gain : Gain  Gain=alt_hold_av  SaturateOnIntegerOverflow=on  OutDataTypeStr=Inherit: Same as input  ParamDataTypeStr=Inherit: Same as input
      settings: AttributesFormatString=%<Gain>
  thetaCmd_rad : Outport  InitialOutput=0
  " qC_rps " : Outport  Port=2  InitialOutput=0
  wires:
  Sum5/1 -> Attitude Gain1/1
  qF_rps/1 -> Outerloop AP Delay/1
  Outerloop AP Delay/1 -> Subsystem1/1(In)
  PFD/MFD Delay2/1 -> Complementary Filter/2(hdd_mpss)
  Vertical Accel Gain/1 -> Sum5/2
  VS Gain/1 -> Sum5/1
  Sum3/1 -> VS Gain/1
  Hold Gain/1 -> Sum3/1
  Subsystem/1(Out) -> thetaCmd_rad/1
  Subsystem1/1(Out) -> " qC_rps "/1
  Complementary Filter/1(hdF_mps) -> Sum3/2
  Complementary Filter/2(hddF_mpss) -> Av_LP/1
  Av_LP/1 -> Vertical Accel Gain/1
  hCmd_m/1 -> Sum1/1
  Sum1/1 -> PFD/MFD Delay/1
  Ground1/1 -> Manual Switch3/1
  Alt Upset_m/1(Signal 2) -> Manual Switch3/2
  Manual Switch3/1 -> Sum2/1
  hF_m/1 -> Sum2/2
  Sum2/1 -> Sum1/2
  Ground2/1 -> Manual Switch1/1
  VS Upset_fpm/1(Signal 2) -> Gain2/1
  Gain2/1 -> Manual Switch1/2
  Sum4/1 -> PFD/MFD Delay1/1
  Manual Switch1/1 -> Sum4/1
  hdF_mps/1 -> Sum4/2
  PFD/MFD Delay/1 -> Hold Gain/1
  PFD/MFD Delay1/1 -> Complementary Filter/1(hd_mps)
  hddF_mpss/1 -> PFD/MFD Delay2/1
  Attitude Gain1/1 -> Outerloop FD Delay/1
  Outerloop FD Delay/1 -> Subsystem/1(In)

== system AFASClosedloopSim/FMGC (Flight Mgt and Guidance & Control)/AFCC: Albatross.ai Flight Control Computer/FCC: Outerloop & Innerloop Control Laws/Autothrottle/ADC Filters & Delays ==
  vtas_mps : Inport
  ADC S/W Filter : TransferFcn  Numerator=[0.0802 1.151 78.01]  Denominator=[1 10.3 78.01]
  ADC S/W and H/W Analog Filter Delay : TransportDelay  DelayTime=0.011
  ARINC429 Delay : TransportDelay  DelayTime=0.047623
  vtasF_mps : Outport
  wires:
  ADC S/W Filter/1 -> ADC S/W and H/W Analog Filter Delay/1
  ADC S/W and H/W Analog Filter Delay/1 -> ARINC429 Delay/1
  ARINC429 Delay/1 -> vtasF_mps/1
  vtas_mps/1 -> ADC S/W Filter/1

== system AFASClosedloopSim/FMGC (Flight Mgt and Guidance & Control)/AFCC: Albatross.ai Flight Control Computer/FCC: Outerloop & Innerloop Control Laws/Autothrottle/AT Innerloop ==
  "ATCmd_rad " : Inport
  Innerloop AT Delay : TransportDelay  DelayTime=0.003
  Lead-Lag : TransferFcn  Numerator=[AT_lead_T1 1]  Denominator=[AT_lead_T2 1]
  Structural Mode Filter3 : TransferFcn  Numerator=AT_struct_num  Denominator=AT_struct_den
  g2mpss2 : Gain  Gain=AT_svo_composite  SaturateOnIntegerOverflow=on  OutDataTypeStr=Inherit: Same as input  ParamDataTypeStr=Inherit: Same as input
  motorPosCmd_rad : Outport  InitialOutput=0
  wires:
  Structural Mode Filter3/1 -> Innerloop AT Delay/1
  "ATCmd_rad "/1 -> g2mpss2/1
  Innerloop AT Delay/1 -> motorPosCmd_rad/1
  g2mpss2/1 -> Lead-Lag/1
  Lead-Lag/1 -> Structural Mode Filter3/1

== system AFASClosedloopSim/FMGC (Flight Mgt and Guidance & Control)/AFCC: Albatross.ai Flight Control Computer/FCC: Outerloop & Innerloop Control Laws/Autothrottle/AT SPD Hold//Select ==
  vtasCmd_mps : Inport
  vtasF_mps : Inport  Port=2
  AT_SPD_LP : TransferFcn  Denominator=[AT_spd_hold_tas_lp_tau 1]
  AT_SPD_LP1 : TransferFcn  Denominator=[AT_spd_hold_tas_val_lp_tau 1]
  AT_spd_hold_cmpst : Gain  Gain=AT_spd_hold_cmpst
  AT_spd_hold_rate_damping_gain : Gain  Gain=AT_spd_hold_rate_damping_gain
  Outerloop FD Delay : TransportDelay  DelayTime=0.0905
  PFD/MFD Delay1 : TransportDelay  DelayTime=0.055
  Subsystem : Subsystem  mask(Zero-Order Hold){Tau=0.100}
      mask prompts: Tau "Tau (s)"
      mask help: Zero-Order Hold
      settings: AttributesFormatString=ZOH\n
      mask Display: disp([num2str(1/Tau),'Hz'])
  Sum1 : Sum  Inputs=|+-  SaturateOnIntegerOverflow=on
  Sum4 : Sum  Inputs=|+-  InputSameDT=on  SaturateOnIntegerOverflow=on  OutDataTypeStr=Inherit: Same as first input
  V_RD_HP : TransferFcn  Numerator="[1   0]"  Denominator="[AT_spd_hold_ptch_tau_gain*tas_mps   1]"
  ATCmd_rad : Outport  InitialOutput=0
  wires:
  V_RD_HP/1 -> AT_spd_hold_rate_damping_gain/1
  AT_spd_hold_rate_damping_gain/1 -> Sum1/2
  Sum1/1 -> AT_spd_hold_cmpst/1
  vtasCmd_mps/1 -> Sum4/1
  PFD/MFD Delay1/1 -> Sum4/2, AT_SPD_LP1/1
  vtasF_mps/1 -> PFD/MFD Delay1/1
  AT_SPD_LP1/1 -> V_RD_HP/1
  AT_spd_hold_cmpst/1 -> Outerloop FD Delay/1
  Sum4/1 -> AT_SPD_LP/1
  Outerloop FD Delay/1 -> Subsystem/1(In)
  AT_SPD_LP/1 -> Sum1/1
  Subsystem/1(Out) -> ATCmd_rad/1

== system AFASClosedloopSim/FMGC (Flight Mgt and Guidance & Control)/AFCC: Albatross.ai Flight Control Computer/FCC: Outerloop & Innerloop Control Laws/HDG Mode/Filters & Delays ==
  psi_rad : Inport
  psiDot_rps : Inport  Port=2
  phi_rad : Inport  Port=3
  phiDot_rps : Inport  Port=4
  rb_rps : Inport  Port=5
  AyAH_mpss : Inport  Port=6
  AHRS Delay{,1..5} (6 alike) : TransportDelay  DelayTime=0.014
  ARINC429 Delay : TransportDelay  DelayTime=0.01225
  ARINC429 Delay1 : TransportDelay  DelayTime=0.00825
  ARINC429 Delay2 : TransportDelay  DelayTime=0.00705
  ARINC429 Delay3 : TransportDelay  DelayTime=0.00785
  ARINC429 Delay4 : TransportDelay  DelayTime=0.00825
  ARINC429 Delay5 : TransportDelay  DelayTime=0.00905
  Ay Anti-aliasing Filter : TransferFcn  Numerator=[2020.20]  Denominator=[1 75.76 2020.20]
  Internal Filter{1..5} (5 alike) : TransferFcn  Numerator=[35600]  Denominator=[1 377.36 35600]
      settings: AttributesFormatString=Internal Filter
  Phi Anti-aliasing Filter : TransferFcn  Numerator=[10000]  Denominator=[1 200 10000]
  PhiDot Anti-aliasing Filter : TransferFcn  Numerator=[10000]  Denominator=[1 200 10000]
  Psi Anti-aliasing Filter : TransferFcn  Numerator=[10000]  Denominator=[1 200 10000]
  PsiDot Anti-aliasing Filter : TransferFcn  Numerator=[10000]  Denominator=[1 200 10000]
  R Anti-aliasing Filter : TransferFcn  Numerator=[10000]  Denominator=[1 200 10000]
  psiF_rad : Outport
  psiDotF_rps : Outport  Port=2
  phiF_rad : Outport  Port=3
  phiDotF_rps : Outport  Port=4
  rF_rps : Outport  Port=5
  AyF_mpss : Outport  Port=6
  wires:
  Psi Anti-aliasing Filter/1 -> AHRS Delay/1
  Internal Filter5/1 -> Psi Anti-aliasing Filter/1
  AHRS Delay2/1 -> ARINC429 Delay2/1
  AHRS Delay3/1 -> ARINC429 Delay3/1
  AHRS Delay4/1 -> ARINC429 Delay4/1
  AHRS Delay5/1 -> ARINC429 Delay5/1
  psi_rad/1 -> Internal Filter5/1
  Internal Filter1/1 -> Phi Anti-aliasing Filter/1
  phi_rad/1 -> Internal Filter1/1
  Phi Anti-aliasing Filter/1 -> AHRS Delay2/1
  Internal Filter2/1 -> PhiDot Anti-aliasing Filter/1
  PhiDot Anti-aliasing Filter/1 -> AHRS Delay3/1
  phiDot_rps/1 -> Internal Filter2/1
  Internal Filter3/1 -> R Anti-aliasing Filter/1
  R Anti-aliasing Filter/1 -> AHRS Delay4/1
  rb_rps/1 -> Internal Filter3/1
  Ay Anti-aliasing Filter/1 -> AHRS Delay5/1
  AyAH_mpss/1 -> Ay Anti-aliasing Filter/1
  ARINC429 Delay2/1 -> phiF_rad/1
  ARINC429 Delay3/1 -> phiDotF_rps/1
  ARINC429 Delay4/1 -> rF_rps/1
  ARINC429 Delay5/1 -> AyF_mpss/1
  psiDot_rps/1 -> Internal Filter4/1
  Internal Filter4/1 -> PsiDot Anti-aliasing Filter/1
  PsiDot Anti-aliasing Filter/1 -> AHRS Delay1/1
  AHRS Delay1/1 -> ARINC429 Delay1/1
  ARINC429 Delay1/1 -> psiDotF_rps/1
  AHRS Delay/1 -> ARINC429 Delay/1
  ARINC429 Delay/1 -> psiF_rad/1

== system AFASClosedloopSim/FMGC (Flight Mgt and Guidance & Control)/AFCC: Albatross.ai Flight Control Computer/FCC: Outerloop & Innerloop Control Laws/HDG Mode/Innerloop Control Law ==
  note: Linear Roll Autopilot & Yaw Damper Model
  phiCmd_rad : Inport
  phiC_rad : Inport  Port=2
  rC_rps : Inport  Port=3
  AyC_mpss : Inport  Port=4
  phidotC_rps : Inport  Port=5
  Gain1 : Gain  Gain=ydEngaged  SaturateOnIntegerOverflow=on  OutDataTypeStr=Inherit: Same as input  ParamDataTypeStr=Inherit: Same as input
      settings: AttributesFormatString=YD On/Off
  Roll AP : Subsystem
  YD Control Law : Subsystem
  ailMotorPosCmd_rad : Outport  InitialOutput=0
  rudMotorPosCmd_rad : Outport  Port=2  InitialOutput=0
  wires:
  Roll AP/1(motorPosCmd_rad) -> ailMotorPosCmd_rad/1
  YD Control Law/1(motorPosCmd_rad) -> Gain1/1
  Gain1/1 -> rudMotorPosCmd_rad/1
  phidotC_rps/1 -> Roll AP/1(phidotC_rps)
  phiC_rad/1 -> Roll AP/2(phiC_rad), YD Control Law/1(phiC_rad)
  phiCmd_rad/1 -> Roll AP/3(phiCmd_rad)
  AyC_mpss/1 -> YD Control Law/3(AyC_mpss)
  rC_rps/1 -> YD Control Law/2(rC_rps)
